simulink model "TGN2_0028_30_24_model"  (R2016a)
settings: Solver=ode3  StartTime=0.0  StopTime=0.3  FixedStep=1e-4  RelTol=1e-3
InitFcn:
  | mbd_pnt_consistency_checks(bdroot(gcs));
model workspace (MAT data in the model file):
  B = 0
  J = 5e-06
  KC = 0.04
  KV = 0.021
  L = 0.00021
  PP = 3
  R = 0.215
settings Model: Creator=admin_aboyer  LastModifiedBy=admin_aboyer
settings DataIOCC: ExternalInput=off  InitialState=off  SaveOutput=off  SignalLogging=off  SaveTime=off
settings OptimizationCC: BlockReduction=off  DefaultParameterBehavior=Inlined  OptimizeModelRefInitCode=on  LifeSpan=1
settings DebuggingCC: InheritedTsInSrcMsg=none  MultiTaskDSMMsg=none  SingleTaskRateTransMsg=error  UnconnectedInputMsg=error  UnconnectedOutputMsg=error  UnconnectedLineMsg=error  UnknownTsInhSupMsg=error
settings HardwareCC: ProdBitPerPointer=32  ProdLargestAtomicInteger=Long  ProdLargestAtomicFloat=Double  ProdEndianess=BigEndian  ProdWordSize=32  ProdHWDeviceType=Motorola PowerPC
settings RTWCC: SystemTargetFile=mbd_pnt.tlc  MakeCommand=mbd_pnt_make_rtw COPY_MDLREF_INCLUDES=0  TemplateMakefile=mbd_pnt.tmf  Description=Model Based Design Toolbox MPC574xP Code Generation Target  GenerateReport=on  IncludeHyperlinkInReport=on  LaunchReport=on  GenerateTraceInfo=on  GenerateTraceReport=on  GenerateTraceReportSl=on  GenerateTraceReportSf=on  GenerateTraceReportEml=on
settings CodeAppCC: ForceParamTrailComments=on  IgnoreCustomStorageClasses=off  OperatorAnnotations=on  SimulinkDataObjDesc=on  SFDataObjDesc=on  MATLABFcnDesc=on  InsertBlockDesc=on  MATLABSourceComments=on
settings STFCustomTargetCC: GenerateSampleERTMain=on  CombineOutputUpdateFcns=on  SuppressErrorStatus=on  ERTCustomFileBanners=on  SupportContinuousTime=off  SupportNonInlinedSFcns=off  MATLABClassNameForMDSCustomization=Simulink.SoftwareTarget.ERTCustomization  GRTInterface=off  SystemTargetFile=mbd_pnt.tlc
settings ERTTargetCC: GenerateSampleERTMain=on  ParMdlRefBuildCompliant=off  CompOptLevelCompliant=off  ConcurrentExecutionCompliant=off  SuppressErrorStatus=on  ERTFirstTimeCompliant=off  ModelStepFunctionPrototypeControlCompliant=off  CPPClassGenCompliant=off  UseToolchainInfoCompliant=off  InlinedParameterPlacement=NonHierarchical  ERTCustomFileTemplate=example_file_process.tlc

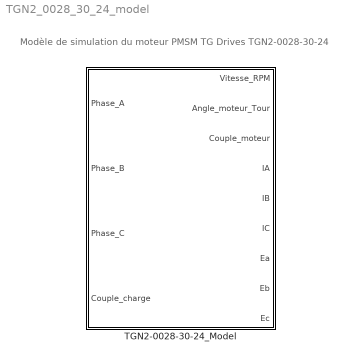
== system TGN2_0028_30_24_model ==
  note: Modèle de simulation du moteur PMSM TG Drives TGN2-0028-30-24
  TGN2-0028-30-24_Model : Subsystem
      mask Display: image('C:\WORKSPACE_MATLAB\PMSM_Workshop\M5\img\PMSM.PNG');

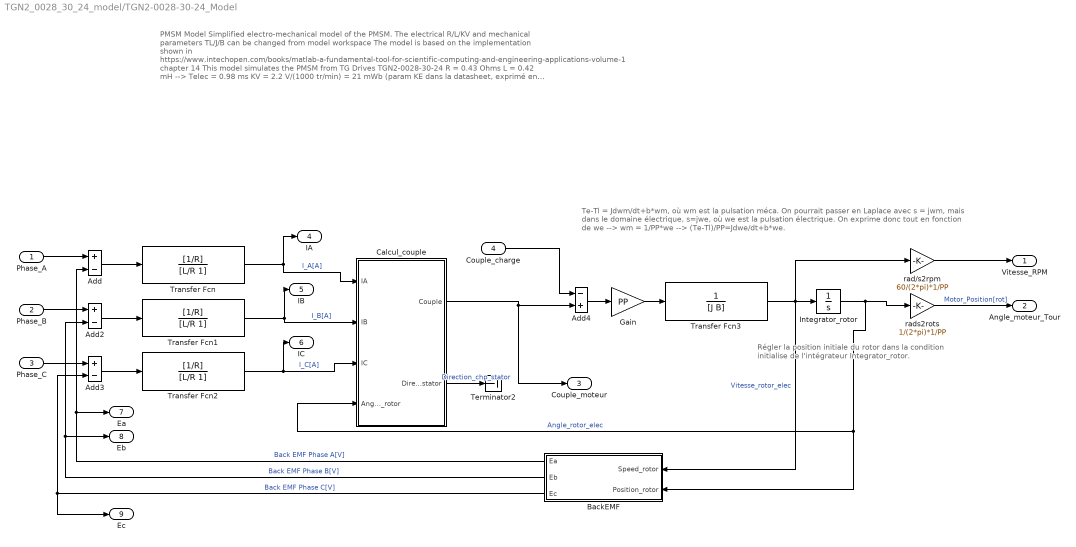
== system TGN2_0028_30_24_model/TGN2-0028-30-24_Model ==
  note: Régler la position initiale du rotor dans la condition
      | initialise de l'intégrateur Integrator_rotor.
  note: Te-Tl = Jdwm/dt+b*wm, où wm est la pulsation méca.
      | On pourrait passer en Laplace avec s = jwm, mais dans le domaine électrique, s=jwe, où we est la pulsation électrique.
      | On exprime donc tout en fonction de we --> wm = 1/PP*we --> (Te-Tl)/PP=Jdwe/dt+b*we.
  note: PMSM Model
      |
      | Simplified electro-mechanical model of the PMSM. The electrical R/L/KV and mechanical parameters TL/J/B can be changed from model workspace
      | The model is based on the implementation shown in https://www.intechopen.com/books/matlab-a-fundamental-tool-for-scientific-computing-and-engineering-applications-volume-1
      | chapter 14
      |
      | This model simulates the PMSM from TG Drives TGN2-0028-30-24
      | R = 0.43 Ohms
      | L = 0.42 mH --> Telec = 0.98 ms
      | KV = 2.2 V/(1000 tr/min) = 21 mWb (param KE dans la datasheet, exprimé en V/(1000x tr.min^1)
      | KC = 40 mNm/A (constante de couple)
      | J = 5e-6 kg*m^2
      | B = 1.79e-3 Nm/rad*s^-1 --> Tmeca = 2.8 ms
      | pp = 1 (pole pairs per phase)
  Phase_A : Inport
  Phase_B : Inport  Port=2
  Phase_C : Inport  Port=3
  Couple_charge : Inport  Port=4
  Add : Sum  Inputs=+-
  Add2 : Sum  Inputs=+-
  Add3 : Sum  Inputs=+-
  Add4 : Sum  Inputs=-+
  BackEMF : Subsystem
  Calcul_couple : Subsystem
  Gain : Gain  Gain=PP
  Integrator_rotor : Integrator  InitialCondition=-pi/2
  Terminator2 : Terminator
  Transfer Fcn : TransferFcn  Numerator=[1/R]  Denominator=[L/R 1]
  Transfer Fcn1 : TransferFcn  Numerator=[1/R]  Denominator=[L/R 1]
  Transfer Fcn2 : TransferFcn  Numerator=[1/R]  Denominator=[L/R 1]
  Transfer Fcn3 : TransferFcn  Denominator=[J B]
  rad/s2rpm : Gain  Gain=60/(2*pi)*1/PP
  rads2rots : Gain  Gain=1/(2*pi)*1/PP
  Vitesse_RPM : Outport
  Angle_moteur_Tour : Outport  Port=2
  Couple_moteur : Outport  Port=3
  IA : Outport  Port=4
  IB : Outport  Port=5
  IC : Outport  Port=6
  Ea : Outport  Port=7
  Eb : Outport  Port=8
  Ec : Outport  Port=9
  wires:
  Add/1 -> Transfer Fcn/1
  Phase_A/1 -> Add/1
  Transfer Fcn/1 -> Calcul_couple/1(IA), IA/1  "I_A[A]"
  Transfer Fcn1/1 -> IB/1, Calcul_couple/2(IB)  "I_B[A]"
  Add2/1 -> Transfer Fcn1/1
  Add3/1 -> Transfer Fcn2/1
  Transfer Fcn2/1 -> IC/1, Calcul_couple/3(IC)  "I_C[A]"
  Phase_B/1 -> Add2/1
  Phase_C/1 -> Add3/1
  Couple_charge/1 -> Add4/1
  Add4/1 -> Gain/1
  Gain/1 -> Transfer Fcn3/1
  Transfer Fcn3/1 -> BackEMF/1(Speed_rotor), rad/s2rpm/1, Integrator_rotor/1  "Vitesse_rotor_elec"
  Calcul_couple/1(Couple) -> Couple_moteur/1, Add4/2
  BackEMF/3(Ec) -> Add3/2, Ec/1  "Back EMF Phase C[V]"
  BackEMF/1(Ea) -> Ea/1, Add/2  "Back EMF Phase A[V]"
  BackEMF/2(Eb) -> Eb/1, Add2/2  "Back EMF Phase B[V]"
  rad/s2rpm/1 -> Vitesse_RPM/1
  Integrator_rotor/1 -> BackEMF/2(Position_rotor), Calcul_couple/4(Angle_rotor), rads2rots/1  "Angle_rotor_elec"
  rads2rots/1 -> Angle_moteur_Tour/1  "Motor_Position[rot]"
  Calcul_couple/2(Direction_Chp_stator) -> Terminator2/1  "Direction_chp_stator"

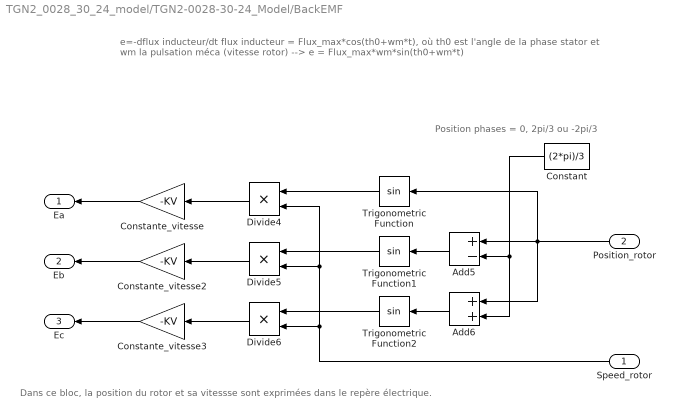
== system TGN2_0028_30_24_model/TGN2-0028-30-24_Model/BackEMF ==
  note: Dans ce bloc, la position du rotor et sa vitessse sont exprimées dans le repère électrique.
  note: e=-dflux inducteur/dt
      | flux inducteur = Flux_max*cos(th0+wm*t), où th0 est l'angle de la phase stator et wm la pulsation méca (vitesse rotor)
      | --> e = Flux_max*wm*sin(th0+wm*t)
  note: Position phases = 0, 2pi/3 ou -2pi/3
  Speed_rotor : Inport
  Position_rotor : Inport  Port=2
  Add5 : Sum  Inputs=+-
  Add6 : Sum
  Constant : Constant  Value=(2*pi)/3
  Constante_vitesse : Gain  Gain=-KV
  Constante_vitesse2 : Gain  Gain=-KV
  Constante_vitesse3 : Gain  Gain=-KV
  Divide4 : Product  Inputs=**
  Divide5 : Product  Inputs=**
  Divide6 : Product  Inputs=**
  Trigonometric Function : Trigonometry
  Trigonometric Function1 : Trigonometry
  Trigonometric Function2 : Trigonometry
  Ea : Outport
  Eb : Outport  Port=2
  Ec : Outport  Port=3
  wires:
  Divide4/1 -> Constante_vitesse/1
  Divide6/1 -> Constante_vitesse3/1
  Trigonometric Function2/1 -> Divide6/1
  Constante_vitesse3/1 -> Ec/1
  Speed_rotor/1 -> Divide4/2, Divide5/2, Divide6/2
  Constante_vitesse2/1 -> Eb/1
  Divide5/1 -> Constante_vitesse2/1
  Constant/1 -> Add6/2, Add5/2
  Add6/1 -> Trigonometric Function2/1
  Trigonometric Function/1 -> Divide4/1
  Add5/1 -> Trigonometric Function1/1
  Constante_vitesse/1 -> Ea/1
  Trigonometric Function1/1 -> Divide5/1
  Position_rotor/1 -> Add5/1, Trigonometric Function/1, Add6/1

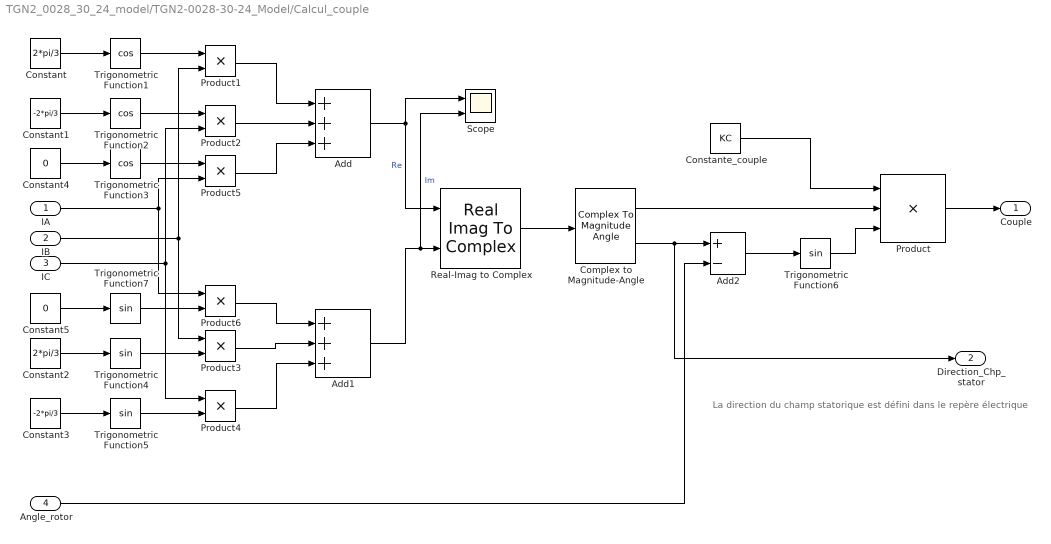
== system TGN2_0028_30_24_model/TGN2-0028-30-24_Model/Calcul_couple ==
  note: La direction du champ statorique est défini dans le repère électrique
  IA : Inport
  IB : Inport  Port=2
  IC : Inport  Port=3
  Angle_rotor : Inport  Port=4
  Add : Sum  Inputs=+++
  Add1 : Sum  Inputs=+++
  Add2 : Sum  Inputs=+-
  Complex to Magnitude-Angle : ComplexToMagnitudeAngle
  Constant : Constant  Value=2*pi/3
  Constant1 : Constant  Value=-2*pi/3
  Constant2 : Constant  Value=2*pi/3
  Constant3 : Constant  Value=-2*pi/3
  Constant4 : Constant  Value=0
  Constant5 : Constant  Value=0
  Constante_couple : Constant  Value=KC
  Product : Product  Inputs=3
  Product{1..6} (6 alike) : Product
  Real-Imag to Complex : RealImagToComplex
  Scope : Scope  NumInputPorts=2
  Trigonometric Function1 : Trigonometry  Operator=cos
  Trigonometric Function2 : Trigonometry  Operator=cos
  Trigonometric Function3 : Trigonometry  Operator=cos
  Trigonometric Function{4..7} (4 alike) : Trigonometry
  Couple : Outport
  Direction_Chp_stator : Outport  Port=2
  wires:
  Add/1 -> Real-Imag to Complex/1, Scope/1  "Re"
  Add1/1 -> Scope/2, Real-Imag to Complex/2  "Im"
  Real-Imag to Complex/1 -> Complex to Magnitude-Angle/1
  Complex to Magnitude-Angle/2 -> Direction_Chp_stator/1, Add2/1
  Angle_rotor/1 -> Add2/2
  Add2/1 -> Trigonometric Function6/1
  Complex to Magnitude-Angle/1 -> Product/2
  Trigonometric Function6/1 -> Product/3
  Constante_couple/1 -> Product/1
  Product/1 -> Couple/1
  Constant1/1 -> Trigonometric Function2/1
  Constant/1 -> Trigonometric Function1/1
  Trigonometric Function1/1 -> Product1/1
  Trigonometric Function2/1 -> Product2/1
  IB/1 -> Product1/2, Product3/1
  IC/1 -> Product4/1, Product2/2
  Product1/1 -> Add/1
  Product2/1 -> Add/2
  Constant3/1 -> Trigonometric Function5/1
  Constant2/1 -> Trigonometric Function4/1
  Trigonometric Function4/1 -> Product3/2
  Trigonometric Function5/1 -> Product4/2
  Product3/1 -> Add1/2
  Product4/1 -> Add1/3
  Constant4/1 -> Trigonometric Function3/1
  Trigonometric Function3/1 -> Product5/1
  IA/1 -> Product6/1, Product5/2
  Product5/1 -> Add/3
  Trigonometric Function7/1 -> Product6/2
  Constant5/1 -> Trigonometric Function7/1
  Product6/1 -> Add1/1
